simulink model "ejemplo_Cyton_alpha"  (R2016a)
settings: Solver=FixedStepAuto  StartTime=0.0  StopTime=inf  FixedStep=0.001  RelTol=1e-3
libraries: simulink x8, LibrarySimulinkSAS x1, aerolibanimutils x1
settings Model: Creator=Usuario  LastModifiedBy=Usuario

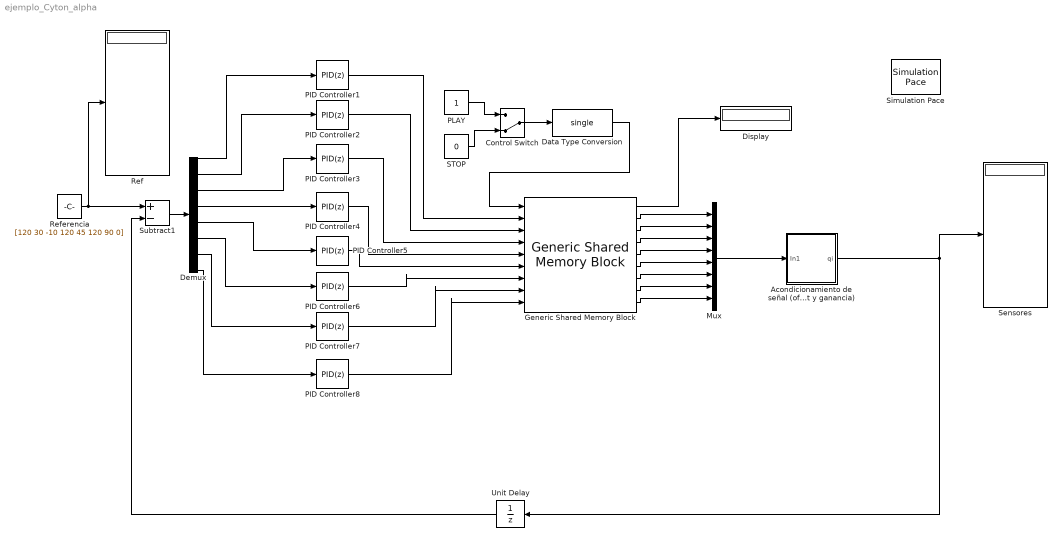
== system ejemplo_Cyton_alpha ==
  Acondicionamiento de señal (offset y ganancia) : Subsystem
  Control Switch : ManualSwitch  CurrentSetting=0
  Data Type Conversion : DataTypeConversion  OutDataTypeStr=single
  Demux : Demux  Outputs=8
  Display : Display
  Generic Shared Memory Block : LibrarySimulinkSAS/Generic Shared Memory Block  nombre='ARDUINO'  dispositivo=1  vecE=[1 1 1 1 1 1 1 1 1]  vecS=[1 1 1 1 1 1 1 1 1]  tipoE=['f' 'f' 'f' 'f' 'f' 'f' 'f' 'f' 'f']  tipoS=['f' 'f' 'f' 'f' 'f' 'f' 'f' 'f' 'f']
  Mux : Mux  Inputs=8
  PID Controller{1..8} (8 alike) : simulink/Continuous/PID Controller  Controller=PID  TimeDomain=Discrete-time  SampleTime=-1  IntegratorMethod=Forward Euler  FilterMethod=Forward Euler  Form=Parallel  UseFilter=on  ControllerParametersSource=internal  P=75  I=40  D=0.01  N=100  InitialConditionSource=internal  InitialConditionForIntegrator=0  InitialConditionForFilter=0  ExternalReset=none  LimitOutput=on  UpperSaturationLimit=4095  LowerSaturationLimit=-4095  LinearizeAsGain=on  AntiWindupMode=clamping  Kb=1  TrackingMode=off  Kt=1  PParamMin=[]  PParamMax=[]  PParamDataTypeStr=single  IParamMin=[]  IParamMax=[]  IParamDataTypeStr=single  DParamMin=[]  DParamMax=[]  DParamDataTypeStr=single  NParamMin=[]  NParamMax=[]  NParamDataTypeStr=single  KbParamMin=[]  KbParamMax=[]  KtParamMin=[]  KtParamMax=[]  POutMin=[]  POutMax=[]  POutDataTypeStr=single  PGainOutDataTypeStr=single  PProdOutDataTypeStr=single  IOutMin=[]  IOutMax=[]  IOutDataTypeStr=single  IGainOutDataTypeStr=single  IProdOutDataTypeStr=single  DOutMin=[]  DOutMax=[]  DOutDataTypeStr=single  DGainOutDataTypeStr=single  DProdOutDataTypeStr=single  NOutMin=[]  NOutMax=[]  NOutDataTypeStr=single  NGainOutDataTypeStr=single  NProdOutDataTypeStr=single  KbOutMin=[]  KbOutMax=[]  KtOutMin=[]  KtOutMax=[]  IntegratorOutMin=[]  IntegratorOutMax=[]  IntegratorOutDataTypeStr=single  FilterOutMin=[]  FilterOutMax=[]  FilterOutDataTypeStr=single  SumOutMin=[]  SumOutMax=[]  SumOutDataTypeStr=single  SumI1OutMin=[]  SumI1OutMax=[]  SumI2OutMin=[]  SumI2OutMax=[]  SumI3OutMin=[]  SumI3OutMax=[]  SumDOutMin=[]  SumDOutMax=[]  SumDOutDataTypeStr=single  SumAccumDataTypeStr=single  SumDAccumDataTypeStr=single  SaturationOutMin=[]  SaturationOutMax=[]  SaturationOutDataTypeStr=single  IntegratorContinuousStateAttributes=''  IntegratorStateMustResolveToSignalObject=off  IntegratorRTWStateStorageClass=Auto  FilterContinuousStateAttributes=''  FilterStateMustResolveToSignalObject=off  FilterRTWStateStorageClass=Auto  DifferentiatorICPrevScaledInput=0  DifferentiatorOutMin=[]  DifferentiatorOutMax=[]
  PLAY : Constant  OutDataTypeStr=single
  Ref : Display
  Referencia : Constant  Value=[120 30 -10 120 45 120 90 0]  OutDataTypeStr=single
  STOP : Constant  Value=0  OutDataTypeStr=single
  Sensores : Display
  Simulation Pace : aerolibanimutils/Simulation Pace  SimulationPace=1  SleepMode=MATLAB Thread  OutputPaceError=off  SampleTime=-1
  Subtract1 : Sum  Inputs=+-
  Unit Delay : UnitDelay  SampleTime=-1
  wires:
  Generic Shared Memory Block/1 -> Display/1
  Generic Shared Memory Block/2 -> Mux/1
  Generic Shared Memory Block/9 -> Mux/8
  Generic Shared Memory Block/7 -> Mux/6
  Generic Shared Memory Block/8 -> Mux/7
  Generic Shared Memory Block/6 -> Mux/5
  Generic Shared Memory Block/3 -> Mux/2
  Generic Shared Memory Block/4 -> Mux/3
  Generic Shared Memory Block/5 -> Mux/4
  Mux/1 -> Acondicionamiento de señal (offset y ganancia)/1(In1)
  Acondicionamiento de señal (offset y ganancia)/1(qi) -> Sensores/1, Unit Delay/1
  PID Controller1/1 -> Generic Shared Memory Block/2
  Unit Delay/1 -> Subtract1/2
  Referencia/1 -> Ref/1, Subtract1/1
  Subtract1/1 -> Demux/1
  Demux/1 -> PID Controller1/1
  Demux/2 -> PID Controller2/1
  PID Controller2/1 -> Generic Shared Memory Block/3
  PID Controller3/1 -> Generic Shared Memory Block/4
  Demux/3 -> PID Controller3/1
  PID Controller4/1 -> Generic Shared Memory Block/5
  Demux/4 -> PID Controller4/1
  PID Controller5/1 -> Generic Shared Memory Block/6
  Demux/5 -> PID Controller5/1
  Demux/6 -> PID Controller6/1
  PID Controller6/1 -> Generic Shared Memory Block/7
  Demux/7 -> PID Controller7/1
  PID Controller7/1 -> Generic Shared Memory Block/8
  PID Controller8/1 -> Generic Shared Memory Block/9
  Demux/8 -> PID Controller8/1
  PLAY/1 -> Control Switch/1
  STOP/1 -> Control Switch/2
  Control Switch/1 -> Data Type Conversion/1
  Data Type Conversion/1 -> Generic Shared Memory Block/1

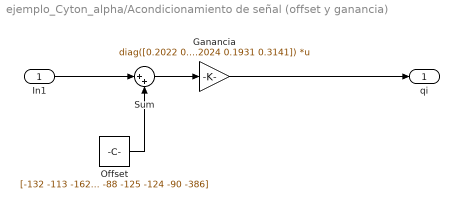
== system ejemplo_Cyton_alpha/Acondicionamiento de señal (offset y ganancia) ==
  In1 : Inport
  Ganancia : Gain  Gain=diag([0.2022 0.2057 0.2093 0.2047 0.2179 0.2024 0.1931 0.3141])  Multiplication=Matrix(K*u) (u vector)
  Offset : Constant  Value=[-132 -113 -162 -88 -125 -124 -90 -386]
  Sum : Sum  Inputs=|++
  qi : Outport
  wires:
  In1/1 -> Sum/1
  Sum/1 -> Ganancia/1
  Offset/1 -> Sum/2
  Ganancia/1 -> qi/1
